simulink model "MinSegPro_Demo"  (R2015a)
settings: Solver=FixedStepDiscrete  SolverMode=SingleTasking  StartTime=0.0  StopTime=inf  FixedStep=.03  RelTol=1e-3
libraries: MinSegLibrary_MinSegPro x4, arduinolib x2, RASPlib x1
settings Model: SimulationMode=external  ExtModeTrigDuration=2  Creator=Alec  LastModifiedBy=hurstj
settings OptimizationCC: ExpressionDepthLimit=2147483647  OptimizeModelRefInitCode=on  LifeSpan=1
settings DebuggingCC: UnderspecifiedInitializationDetection=Classic  MergeDetectMultiDrivingBlocksExec=none  StateNameClashWarn=warning
settings HardwareCC: ProdBitPerInt=16  ProdBitPerPointer=8  ProdIntDivRoundTo=Zero  ProdEndianess=LittleEndian  ProdWordSize=8  ProdHWDeviceType=Atmel->AVR
settings RTWCC: SystemTargetFile=realtime.tlc  GenerateMakefile=off  TemplateMakefile=realtime.tmf  Description=Real-Time Toolbox  RTWVerbose=off
settings CodeAppCC: CustomSymbolStrType=$N$R$M  InternalIdentifier=Classic
settings ERTTargetCC: CombineOutputUpdateFcns=off  ExtMode=on  ExtModeTransport=3  ExtModeMexArgs=0 45 115200 30  ERTSrcFileBannerTemplate=realtime_code_template.cgt  ERTHdrFileBannerTemplate=realtime_code_template.cgt  ERTDataSrcFileTemplate=realtime_code_template.cgt  ERTDataHdrFileTemplate=realtime_code_template.cgt  ERTCustomFileTemplate=realtime_file_process.tlc

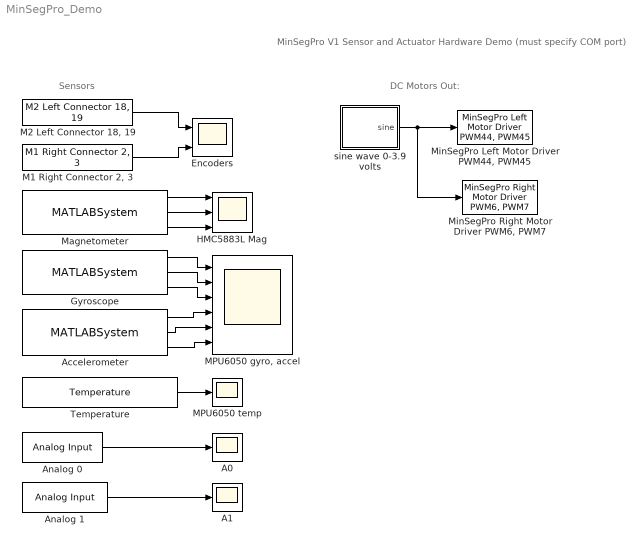
== system MinSegPro_Demo ==
  note: MinSegPro V1 Sensor and Actuator
      | Hardware Demo (must specify COM port)
  note: DC Motors Out:
  note: Sensors
  "A0 " : Scope
      settings: TimeRange=30  YMin=100  YMax=1100  SaveName=ScopeData3
  A1 : Scope
      settings: TimeRange=30  YMin=300  YMax=1100  SaveName=ScopeData4
  Accelerometer : MATLABSystem  System=soMPU6050Accel  SimulateUsing=Code generation
      mask Type: soMPU6050Accel
      mask Display:
      | disp('soMPU6050Accel');
      | port_label('output',1,'xaccel');
      | port_label('output',2,'yaccel');
      | port_label('output',3,'zaccel');
  Analog 0 : arduinolib/Analog Input  pinNumber=0  sampleTime=-1  blockPlatform=arduino
  Analog 1 : arduinolib/Analog Input  pinNumber=1  sampleTime=-1  blockPlatform=arduino
  Encoders : Scope  NumInputPorts=2
      settings: TimeRange=30  YMin=-300~-350  YMax=150~25
  Gyroscope : MATLABSystem  System=soMPU6050Gyro  DLPFmode=0
      mask Type: soMPU6050Gyro
      mask Display:
      | disp('soMPU6050Gyro');
      | port_label('output',1,'xvel');
      | port_label('output',2,'yvel');
      | port_label('output',3,'zvel');
  HMC5883L Mag : Scope  NumInputPorts=3
      settings: TimeRange=10  YMin=-500~450~275  YMax=-300~775~550  SaveName=ScopeData7
  "M1 Right Connector 2, 3" : MinSegLibrary_MinSegPro/M1 Right Connector 2, 3  Encoder=0  PinA=2  PinB=3  PWMFSelect=3  PWMTimer=-1
  "M2 Left Connector 18, 19" : MinSegLibrary_MinSegPro/M2 Left Connector 18, 19  Encoder=1  PinA=19  PinB=18  PWMFSelect=3  PWMTimer=-1
  "MPU6050 gyro, accel" : Scope  NumInputPorts=6
      settings: TimeRange=10  YMin=-40000~-40000~-40000~-12500~-8000~7500  YMax=40000~40000~40000~5000~3000~27500
  MPU6050 temp : Scope
      settings: TimeRange=30  YMin=-3750  YMax=-1750  SaveName=ScopeData2
  Magnetometer : MATLABSystem  System=soHMC5883L  SimulateUsing=Code generation
      mask Type: soHMC5883L
      mask Display:
      | disp('soHMC5883L');
      | port_label('output',1,'xmag');
      | port_label('output',2,'ymag');
      | port_label('output',3,'zmag');
  "MinSegPro Left Motor Driver PWM44, PWM45" : MinSegLibrary_MinSegPro/MinSegPro Left Motor Driver PWM44, PWM45  Vsupply=3.9  PWMoffset=0
  "MinSegPro Right Motor Driver PWM6, PWM7 " : MinSegLibrary_MinSegPro/MinSegPro Right Motor Driver PWM6, PWM7   Vsupply=3.9  PWMoffset=0
  Temperature : RASPlib/Temperature  SimulateUsing=Code generation
  sine wave 0-3.9 volts : Subsystem
  wires:
  sine wave 0-3.9 volts/1(sine) -> "MinSegPro Right Motor Driver PWM6, PWM7 "/1, "MinSegPro Left Motor Driver PWM44, PWM45"/1
  Analog 0/1 -> "A0 "/1
  Analog 1/1 -> A1/1
  Magnetometer/2 -> HMC5883L Mag/2
  Magnetometer/3 -> HMC5883L Mag/3
  Magnetometer/1 -> HMC5883L Mag/1
  Gyroscope/1 -> "MPU6050 gyro, accel"/1
  Gyroscope/2 -> "MPU6050 gyro, accel"/2
  Gyroscope/3 -> "MPU6050 gyro, accel"/3
  Accelerometer/3 -> "MPU6050 gyro, accel"/6
  Accelerometer/2 -> "MPU6050 gyro, accel"/5
  Accelerometer/1 -> "MPU6050 gyro, accel"/4
  "M2 Left Connector 18, 19"/1 -> Encoders/1
  "M1 Right Connector 2, 3"/1 -> Encoders/2
  Temperature/1 -> MPU6050 temp/1

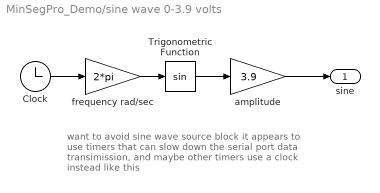
== system MinSegPro_Demo/sine wave 0-3.9 volts ==
  note: want to avoid sine wave source block
      | it appears to use timers that can slow down the
      | serial port data transimission, and maybe
      | other timers
      |
      | use a clock instead like this
  Clock : Clock
  Trigonometric Function : Trigonometry
  amplitude : Gain  Gain=3.9
  frequency rad/sec : Gain  Gain=2*pi
  sine : Outport
  wires:
  amplitude/1 -> sine/1
  frequency rad/sec/1 -> Trigonometric Function/1
  Trigonometric Function/1 -> amplitude/1
  Clock/1 -> frequency rad/sec/1
